simulink model "realtimeE1"  (R2024b)
settings: Solver=FixedStepDiscrete  StartTime=0.0  StopTime=10.0  FixedStep=0.01  RelTol=1e-3  EnableMultiTasking=on
values from neighbouring files (symbols this model uses):
  C = [1,0,0,0]    [S6S10.m]
  CCC = Ts/(Tc+Ts)    [S6S10.m]
undefined symbols (not defined in the file or in its folder): denFd, denH, denHw, DiscIntNeverNeededParam, drv, dspblkCoreblockFVToolHelper, gbox, gcbh, integral, K, numFd, numH, numHw, sens, Ts, wheel
libraries: BalRobTbx_baselib x9
settings Model: ExtModeTrigDuration=2  Creator=lucag  LastModifiedBy=galeazzolu
settings SolverCC: AutoInsertRateTranBlk=on
settings OptimizationCC: EnhancedBackFolding=on  PassReuseOutputArgsAs=Individual arguments  ZeroExternalMemoryAtStartup=off  ZeroInternalMemoryAtStartup=off  MaxStackSize=64  OptimizeBlockOrder=speed  DifferentSizesBufferReuse=on  OptimizationCustomize=off  EfficientTunableParamExpr=on
settings DebuggingCC: ParameterTunabilityLossMsg=error
settings HardwareCC: ProdBitPerInt=16  ProdBitPerPointer=16  ProdBitPerSizeT=16  ProdBitPerPtrDiffT=16  ProdLargestAtomicFloat=None  ProdWordSize=8  ProdHWDeviceType=Atmel->AVR
settings SFSimCC: MATLABDynamicMemAlloc=off
settings RTWCC: Description=Embedded Coder  SystemTargetFile=ert.tlc  HardwareBoard=Arduino Mega 2560  TemplateMakefile=ert_default_tmf  Toolchain=Arduino AVR  BuildConfiguration=Faster Runs
settings CodeAppCC: ForceParamTrailComments=on  IgnoreCustomStorageClasses=off  OperatorAnnotations=on  SimulinkDataObjDesc=on  SFDataObjDesc=on  InsertBlockDesc=on
settings ERTTargetCC: SupportContinuousTime=on  SupportVariableSizeSignals=on  ExtModeTransport=3  ExtModeStaticAlloc=on  ExtModeAutomaticAllocSize=off  ExtModeStaticAllocSize=2048  ExtModeMexFile=ext_xcp  ExtModeIntrfLevel=Level2 - Open  InlinedParameterPlacement=Hierarchical

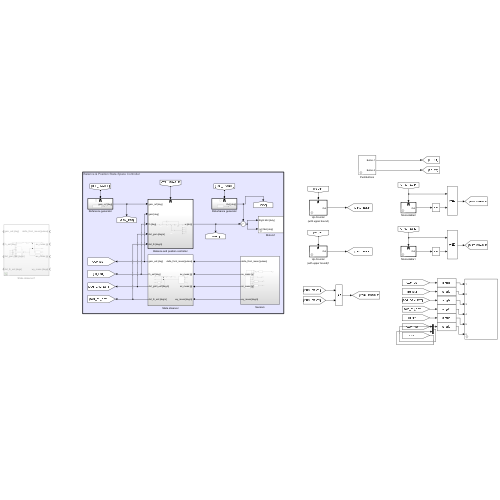
[thumbnail: Simulink's stored preview of the top-level diagram]
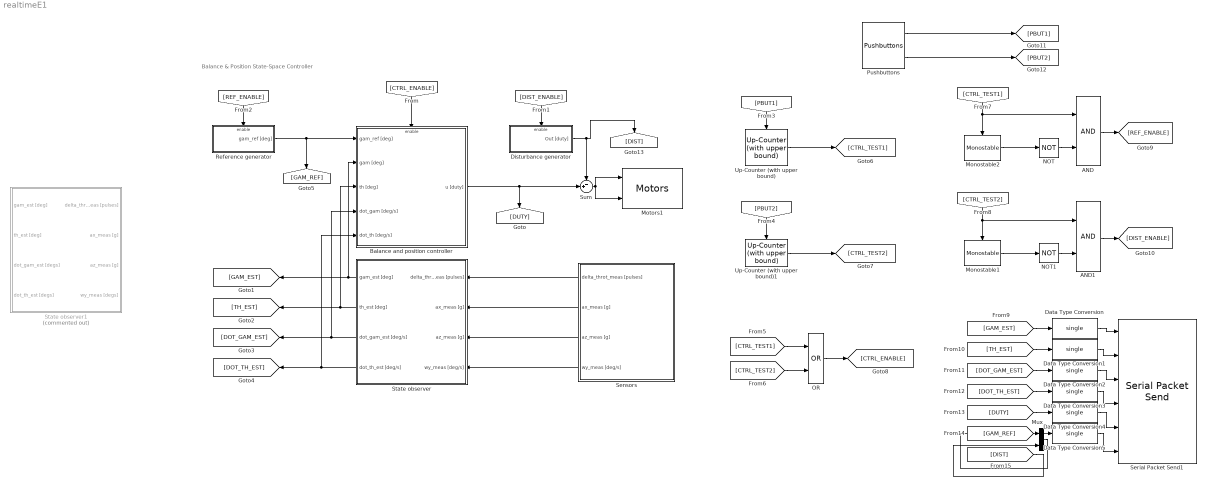
== system realtimeE1 ==
  note: Balance & Position State-Space Controller
  AND : Logic  AllPortsSameDT=off  OutDataTypeStr=boolean
  AND1 : Logic  AllPortsSameDT=off  OutDataTypeStr=boolean
  Balance and position controller : Subsystem  TreatAsAtomicUnit=on
  Data Type Conversion{,1..5} (6 alike) : DataTypeConversion  OutDataTypeStr=single  SaturateOnIntegerOverflow=off  RndMeth=Floor
  Disturbance generator : Subsystem  TreatAsAtomicUnit=on
  Monostable1 : BalRobTbx_baselib/Utilities/Monostable  Tp=13
      settings: SourceProductName=Balancing Robot Toolbox
  Monostable2 : BalRobTbx_baselib/Utilities/Monostable  Tp=10
      settings: SourceProductName=Balancing Robot Toolbox
  Motors1 : BalRobTbx_baselib/Outputs/Motors
      settings: SourceProductName=Balancing Robot Toolbox
  Mux : Mux  Inputs=2
  NOT : Logic  Operator=NOT  AllPortsSameDT=off  OutDataTypeStr=boolean
  NOT1 : Logic  Operator=NOT  AllPortsSameDT=off  OutDataTypeStr=boolean
  OR : Logic  Operator=OR  AllPortsSameDT=off  OutDataTypeStr=boolean
  Pushbuttons : BalRobTbx_baselib/Inputs/Pushbuttons
      settings: SourceProductName=Balancing Robot Toolbox
  Reference generator : Subsystem  TreatAsAtomicUnit=on
  Sensors : Subsystem
  Serial Packet Send1 : BalRobTbx_baselib/Communication/Serial Packet Send  serialLinkOpt=Bluetooth  baudRateOpt=38400  waitHostTxCmd=on  txStartCmd=65  txStopCmd=66  packetSpec={'single', 'single', 'single', 'single', 'single', '2*single'}  cobsEncoded=on  nullTerminated=on  showEnablePort=off
      settings: SourceProductName=Balancing Robot Toolbox
  State observer : Subsystem
  State observer1 : Subsystem  Commented=on
  Sum : Sum  Inputs=-+|
  Up-Counter (with upper bound) : BalRobTbx_baselib/Utilities/Up-Counter (with upper bound)  CMAX=1  C0=0
      settings: SourceProductName=Balancing Robot Toolbox
  Up-Counter (with upper bound)1 : BalRobTbx_baselib/Utilities/Up-Counter (with upper bound)  CMAX=1  C0=0
      settings: SourceProductName=Balancing Robot Toolbox
  wires:
  [CTRL_ENABLE] -> Balance and position controller/Enable
  Balance and position controller/1(u [duty]) -> [DUTY], Sum/2
  Disturbance generator/1(Out [duty]) -> [DIST], Sum/1
  [DIST_ENABLE] -> Disturbance generator/Enable
  Sum/1 -> Motors1/1, Motors1/2
  Sensors/1(delta_throt_meas [pulses]) -> State observer/1(delta_throt_meas [pulses])
  Sensors/2(ax_meas [g]) -> State observer/2(ax_meas [g])
  Sensors/3(az_meas [g]) -> State observer/3(az_meas [g])
  Sensors/4(wy_meas [deg/s]) -> State observer/4(wy_meas [deg/s])
  State observer/1(gam_est [deg]) -> Balance and position controller/2(gam [deg]), [GAM_EST]
  State observer/2(th_est [deg]) -> Balance and position controller/3(th [deg]), [TH_EST]
  State observer/3(dot_gam_est [deg/s]) -> Balance and position controller/4(dot_gam [deg/s]), [DOT_GAM_EST]
  State observer/4(dot_th_est [deg/s]) -> Balance and position controller/5(dot_th [deg/s]), [DOT_TH_EST]
  Reference generator/1(gam_ref [deg]) -> Balance and position controller/1(gam_ref [deg]), [GAM_REF]
  [REF_ENABLE] -> Reference generator/Enable
  [PBUT1] -> Up-Counter (with upper bound)/Trigger
  Up-Counter (with upper bound)/1 -> [CTRL_TEST1]
  Up-Counter (with upper bound)1/1 -> [CTRL_TEST2]
  [PBUT2] -> Up-Counter (with upper bound)1/Trigger
  [CTRL_TEST1] -> OR/1
  [CTRL_TEST2] -> OR/2
  OR/1 -> [CTRL_ENABLE]
  [CTRL_TEST1] -> Monostable2/Enable, AND/1
  Monostable2/1 -> NOT/1
  NOT/1 -> AND/2
  AND/1 -> [REF_ENABLE]
  AND1/1 -> [DIST_ENABLE]
  NOT1/1 -> AND1/2
  Monostable1/1 -> NOT1/1
  Pushbuttons/2 -> [PBUT2]
  Pushbuttons/1 -> [PBUT1]
  [CTRL_TEST2] -> Monostable1/Enable, AND1/1
  [GAM_EST] -> Data Type Conversion/1
  [TH_EST] -> Data Type Conversion1/1
  [DOT_GAM_EST] -> Data Type Conversion2/1
  [DOT_TH_EST] -> Data Type Conversion3/1
  [DUTY] -> Data Type Conversion4/1
  Data Type Conversion5/1 -> Serial Packet Send1/6
  Data Type Conversion4/1 -> Serial Packet Send1/5
  Data Type Conversion3/1 -> Serial Packet Send1/4
  Data Type Conversion2/1 -> Serial Packet Send1/3
  Data Type Conversion1/1 -> Serial Packet Send1/2
  Data Type Conversion/1 -> Serial Packet Send1/1
  [GAM_REF] -> Mux/1
  [DIST] -> Mux/2
  Mux/1 -> Data Type Conversion5/1

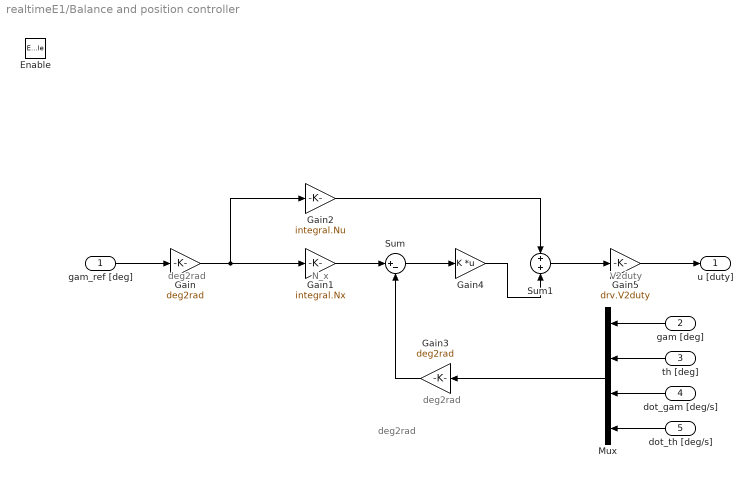
== system realtimeE1/Balance and position controller ==
  note: deg2rad
  note: deg2rad
  note: deg2rad
  note: N_x
  note: V2duty
  gam_ref [deg] : Inport
  gam [deg] : Inport  Port=2
  th [deg] : Inport  Port=3
  dot_gam [deg/s] : Inport  Port=4
  dot_th [deg/s] : Inport  Port=5
  Enable : EnablePort
  Gain : Gain  Gain=deg2rad
  Gain1 : Gain  Gain=integral.Nx
  Gain2 : Gain  Gain=integral.Nu
  Gain3 : Gain  Gain=deg2rad
  Gain4 : Gain  Gain=K  Multiplication=Matrix(K*u)
  Gain5 : Gain  Gain=drv.V2duty
  Mux : Mux
  Sum : Sum  Inputs=|+-
  Sum1 : Sum
  u [duty] : Outport
  wires:
  th [deg]/1 -> Mux/2
  Gain1/1 -> Sum/1
  Gain5/1 -> u [duty]/1
  Gain/1 -> Gain2/1, Gain1/1
  Gain2/1 -> Sum1/1
  Gain3/1 -> Sum/2
  Sum/1 -> Gain4/1
  Mux/1 -> Gain3/1
  Gain4/1 -> Sum1/2
  gam [deg]/1 -> Mux/1
  Sum1/1 -> Gain5/1
  dot_th [deg/s]/1 -> Mux/4
  gam_ref [deg]/1 -> Gain/1
  dot_gam [deg/s]/1 -> Mux/3

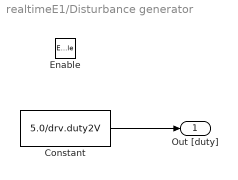
== system realtimeE1/Disturbance generator ==
  Enable : EnablePort
  Constant : Constant  Value=5.0/drv.duty2V
  Out [duty] : Outport  OutputWhenDisabled=reset  InitialOutput=0
  wires:
  Constant/1 -> Out [duty]/1

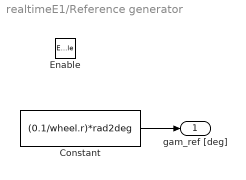
== system realtimeE1/Reference generator ==
  Enable : EnablePort
  Constant : Constant  Value=(0.1/wheel.r)*rad2deg
  gam_ref [deg] : Outport  OutputWhenDisabled=reset  InitialOutput=0
  wires:
  Constant/1 -> gam_ref [deg]/1

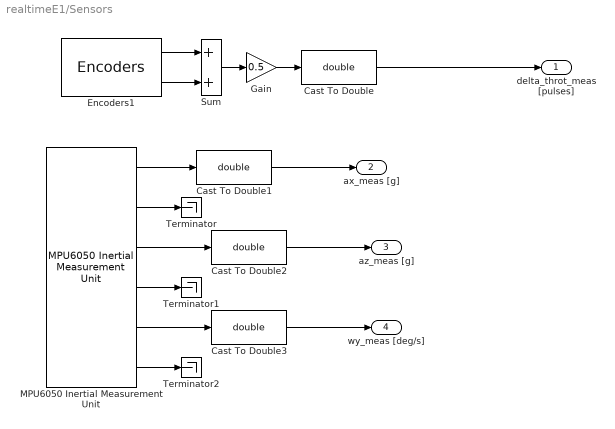
== system realtimeE1/Sensors ==
  Cast To Double{,1..3} (4 alike) : DataTypeConversion  OutDataTypeStr=double  SaturateOnIntegerOverflow=off  RndMeth=Floor
  Encoders1 : BalRobTbx_baselib/Inputs/Encoders
      settings: SourceProductName=Balancing Robot Toolbox
  Gain : Gain  Gain=0.5
  MPU6050 Inertial Measurement Unit : BalRobTbx_baselib/Inputs/MPU6050 Inertial Measurement Unit
      settings: SourceProductName=Balancing Robot Toolbox
  Sum : Sum
  Terminator : Terminator
  Terminator1 : Terminator
  Terminator2 : Terminator
  delta_throt_meas [pulses] : Outport
  ax_meas [g] : Outport  Port=2
  az_meas [g] : Outport  Port=3
  wy_meas [deg/s] : Outport  Port=4
  wires:
  Encoders1/1 -> Sum/1
  Encoders1/2 -> Sum/2
  Sum/1 -> Gain/1
  Gain/1 -> Cast To Double/1
  Cast To Double/1 -> delta_throt_meas [pulses]/1
  MPU6050 Inertial Measurement Unit/1 -> Cast To Double1/1
  MPU6050 Inertial Measurement Unit/3 -> Cast To Double2/1
  MPU6050 Inertial Measurement Unit/5 -> Cast To Double3/1
  MPU6050 Inertial Measurement Unit/2 -> Terminator/1
  MPU6050 Inertial Measurement Unit/4 -> Terminator1/1
  MPU6050 Inertial Measurement Unit/6 -> Terminator2/1
  Cast To Double1/1 -> ax_meas [g]/1
  Cast To Double2/1 -> az_meas [g]/1
  Cast To Double3/1 -> wy_meas [deg/s]/1

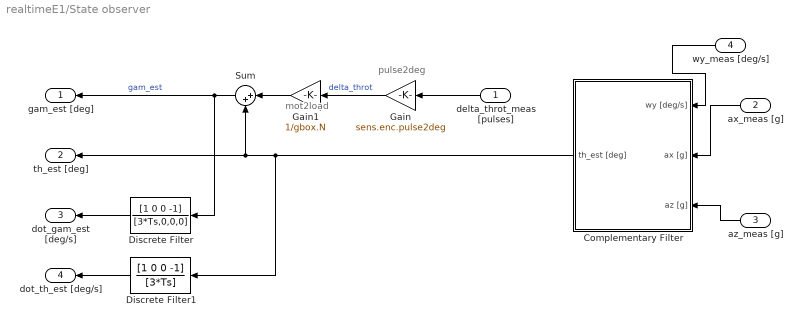
== system realtimeE1/State observer ==
  note: mot2load
  note: pulse2deg
  delta_throt_meas [pulses] : Inport
  ax_meas [g] : Inport  Port=2
  az_meas [g] : Inport  Port=3
  wy_meas [deg/s] : Inport  Port=4
  Complementary Filter : Subsystem
  Discrete Filter : DiscreteFilter  LoadFcn=dspblkCoreblockFVToolHelper(gcbh,'load');  Numerator=[1 0 0 -1]  Denominator=[3*Ts,0,0,0]  SampleTime=Ts
      settings: CopyFcn=dspblkCoreblockFVToolHelper(gcbh,'copy');  DeleteFcn=dspblkCoreblockFVToolHelper(gcbh,'close');  ModelCloseFcn=dspblkCoreblockFVToolHelper(gcbh,'close');  PreSaveFcn=dspblkCoreblockFVToolHelper(gcbh,'presave');  PostSaveFcn=dspblkCoreblockFVToolHelper(gcbh,'postsave');  CloseFcn=dspblkCoreblockFVToolHelper(gcbh,'close');
  Discrete Filter1 : DiscreteFilter  LoadFcn=dspblkCoreblockFVToolHelper(gcbh,'load');  Numerator=[1 0 0 -1]  Denominator=[3*Ts]  SampleTime=Ts
      settings: CopyFcn=dspblkCoreblockFVToolHelper(gcbh,'copy');  DeleteFcn=dspblkCoreblockFVToolHelper(gcbh,'close');  ModelCloseFcn=dspblkCoreblockFVToolHelper(gcbh,'close');  PreSaveFcn=dspblkCoreblockFVToolHelper(gcbh,'presave');  PostSaveFcn=dspblkCoreblockFVToolHelper(gcbh,'postsave');  CloseFcn=dspblkCoreblockFVToolHelper(gcbh,'close');
  Gain : Gain  Gain=sens.enc.pulse2deg
  Gain1 : Gain  Gain=1/gbox.N
  Sum : Sum  Inputs=|++
  gam_est [deg] : Outport
  th_est [deg] : Outport  Port=2
  dot_gam_est [deg/s] : Outport  Port=3
  dot_th_est [deg/s] : Outport  Port=4
  wires:
  Discrete Filter1/1 -> dot_th_est [deg/s]/1
  Sum/1 -> Discrete Filter/1, gam_est [deg]/1  "gam_est"
  Complementary Filter/1(th_est [deg]) -> Discrete Filter1/1, Sum/2, th_est [deg]/1
  Gain1/1 -> Sum/1
  delta_throt_meas [pulses]/1 -> Gain/1
  Discrete Filter/1 -> dot_gam_est [deg/s]/1
  Gain/1 -> Gain1/1  "delta_throt"
  az_meas [g]/1 -> Complementary Filter/3(az [g])
  wy_meas [deg/s]/1 -> Complementary Filter/1(wy [deg/s])
  ax_meas [g]/1 -> Complementary Filter/2(ax [g])

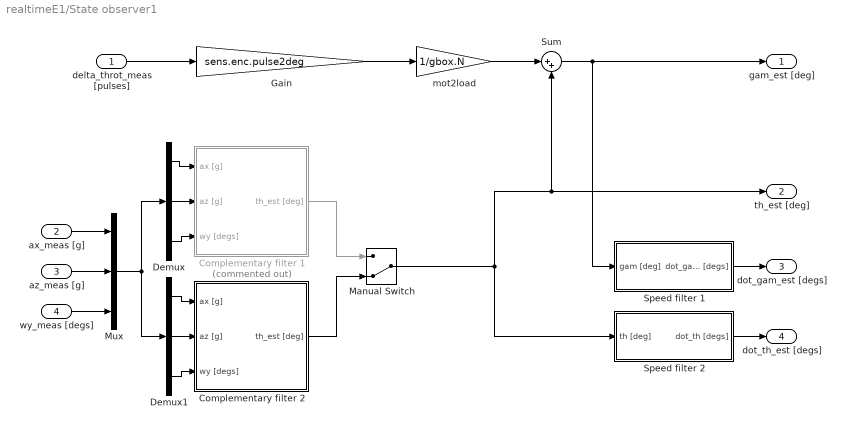
== system realtimeE1/State observer1 ==
  delta_throt_meas [pulses] : Inport
  ax_meas [g] : Inport  Port=2
  az_meas [g] : Inport  Port=3
  wy_meas [degs] : Inport  Port=4
  Complementary filter 1 : Subsystem  Commented=on
  Complementary filter 2 : Subsystem
  Demux : Demux  Outputs=3
  Demux1 : Demux  Outputs=3
  Gain : Gain  Gain=sens.enc.pulse2deg
  Manual Switch : ManualSwitch  CurrentSetting=0
  Mux : Mux  Inputs=3
  Speed filter 1 : Subsystem
  Speed filter 2 : Subsystem
  Sum : Sum  Inputs=|++
  mot2load : Gain  Gain=1/gbox.N
  gam_est [deg] : Outport
  th_est [deg] : Outport  Port=2
  dot_gam_est [degs] : Outport  Port=3
  dot_th_est [degs] : Outport  Port=4
  wires:
  delta_throt_meas [pulses]/1 -> Gain/1
  Gain/1 -> mot2load/1
  mot2load/1 -> Sum/1
  Sum/1 -> Speed filter 1/1(gam [deg]), gam_est [deg]/1
  Speed filter 1/1(dot_gam [degs]) -> dot_gam_est [degs]/1
  Speed filter 2/1(dot_th [degs]) -> dot_th_est [degs]/1
  ax_meas [g]/1 -> Mux/1
  az_meas [g]/1 -> Mux/2
  wy_meas [degs]/1 -> Mux/3
  Demux/1 -> Complementary filter 1/1(ax [g])
  Demux/3 -> Complementary filter 1/3(wy [degs])
  Demux/2 -> Complementary filter 1/2(az [g])
  Demux1/2 -> Complementary filter 2/2(az [g])
  Demux1/1 -> Complementary filter 2/1(ax [g])
  Demux1/3 -> Complementary filter 2/3(wy [degs])
  Mux/1 -> Demux/1, Demux1/1
  Complementary filter 1/1(th_est [deg]) -> Manual Switch/1
  Complementary filter 2/1(th_est [deg]) -> Manual Switch/2
  Manual Switch/1 -> Sum/2, th_est [deg]/1, Speed filter 2/1(th [deg])

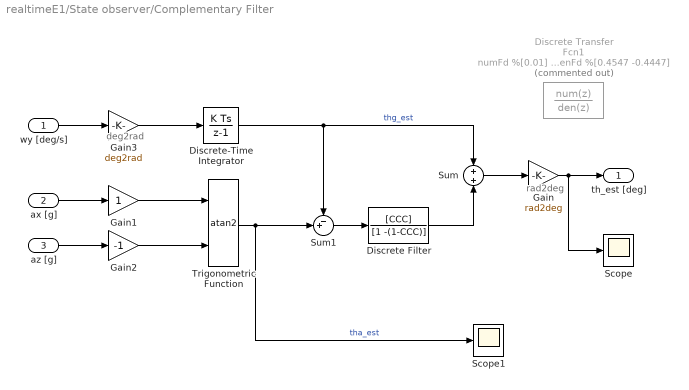
== system realtimeE1/State observer/Complementary Filter ==
  note: rad2deg
  note: deg2rad
  wy [deg/s] : Inport
  ax [g] : Inport  Port=2
  az [g] : Inport  Port=3
  Discrete Transfer Fcn1 : DiscreteTransferFcn  Commented=on  LoadFcn=dspblkCoreblockFVToolHelper(gcbh,'load');  Numerator=numFd %[0.01]  Denominator=denFd %[0.4547 -0.4447]  SampleTime=Ts
      settings: CopyFcn=dspblkCoreblockFVToolHelper(gcbh,'copy');  DeleteFcn=dspblkCoreblockFVToolHelper(gcbh,'close');  ModelCloseFcn=dspblkCoreblockFVToolHelper(gcbh,'close');  PreSaveFcn=dspblkCoreblockFVToolHelper(gcbh,'presave');  PostSaveFcn=dspblkCoreblockFVToolHelper(gcbh,'postsave');  CloseFcn=dspblkCoreblockFVToolHelper(gcbh,'close');
  Discrete Filter : DiscreteFilter  LoadFcn=dspblkCoreblockFVToolHelper(gcbh,'load');  Numerator=[CCC]  Denominator=[1 -(1-CCC)]
      settings: CopyFcn=dspblkCoreblockFVToolHelper(gcbh,'copy');  DeleteFcn=dspblkCoreblockFVToolHelper(gcbh,'close');  ModelCloseFcn=dspblkCoreblockFVToolHelper(gcbh,'close');  PreSaveFcn=dspblkCoreblockFVToolHelper(gcbh,'presave');  PostSaveFcn=dspblkCoreblockFVToolHelper(gcbh,'postsave');  CloseFcn=dspblkCoreblockFVToolHelper(gcbh,'close');
  Discrete-Time Integrator : DiscreteIntegrator  SampleTime=Ts  ICPrevOutput=DiscIntNeverNeededParam  ICPrevScaledInput=DiscIntNeverNeededParam
  Gain : Gain  Gain=rad2deg
  Gain1 : Gain
  Gain2 : Gain  Gain=-1
  Gain3 : Gain  Gain=deg2rad
  Scope : Scope
  Scope1 : Scope
  Sum : Sum  Inputs=+|+
  Sum1 : Sum  Inputs=-+|
  Trigonometric Function : Trigonometry  Operator=atan2
  th_est [deg] : Outport
  wires:
  Sum/1 -> Gain/1
  ax [g]/1 -> Gain1/1
  Gain1/1 -> Trigonometric Function/1
  az [g]/1 -> Gain2/1
  Gain2/1 -> Trigonometric Function/2
  wy [deg/s]/1 -> Gain3/1
  Gain3/1 -> Discrete-Time Integrator/1
  Trigonometric Function/1 -> Scope1/1, Sum1/2  "tha_est"
  Discrete-Time Integrator/1 -> Sum/1, Sum1/1  "thg_est"
  Sum1/1 -> Discrete Filter/1
  Discrete Filter/1 -> Sum/2
  Gain/1 -> Scope/1, th_est [deg]/1

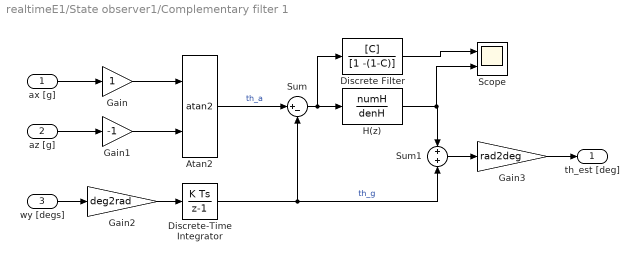
== system realtimeE1/State observer1/Complementary filter 1 ==
  ax [g] : Inport
  az [g] : Inport  Port=2
  wy [degs] : Inport  Port=3
  Atan2 : Trigonometry  Operator=atan2
  Discrete Filter : DiscreteFilter  LoadFcn=dspblkCoreblockFVToolHelper(gcbh,'load');  Numerator=[C]  Denominator=[1 -(1-C)]
      settings: CopyFcn=dspblkCoreblockFVToolHelper(gcbh,'copy');  DeleteFcn=dspblkCoreblockFVToolHelper(gcbh,'close');  ModelCloseFcn=dspblkCoreblockFVToolHelper(gcbh,'close');  PreSaveFcn=dspblkCoreblockFVToolHelper(gcbh,'presave');  PostSaveFcn=dspblkCoreblockFVToolHelper(gcbh,'postsave');  CloseFcn=dspblkCoreblockFVToolHelper(gcbh,'close');
  Discrete-Time Integrator : DiscreteIntegrator  SampleTime=Ts  ICPrevOutput=DiscIntNeverNeededParam  ICPrevScaledInput=DiscIntNeverNeededParam
  Gain : Gain
  Gain1 : Gain  Gain=-1
  Gain2 : Gain  Gain=deg2rad
  Gain3 : Gain  Gain=rad2deg
  H(z) : DiscreteTransferFcn  Numerator=numH  Denominator=denH
  Scope : Scope  NumInputPorts=2
  Sum : Sum  Inputs=|+-
  Sum1 : Sum  Inputs=+|+
  th_est [deg] : Outport
  wires:
  ax [g]/1 -> Gain/1
  az [g]/1 -> Gain1/1
  Gain/1 -> Atan2/1
  Gain1/1 -> Atan2/2
  Atan2/1 -> Sum/1  "th_a"
  wy [degs]/1 -> Gain2/1
  Gain2/1 -> Discrete-Time Integrator/1
  Discrete-Time Integrator/1 -> Sum1/2, Sum/2  "th_g"
  Sum/1 -> Discrete Filter/1, H(z)/1
  H(z)/1 -> Scope/2, Sum1/1
  Sum1/1 -> Gain3/1
  Gain3/1 -> th_est [deg]/1
  Discrete Filter/1 -> Scope/1

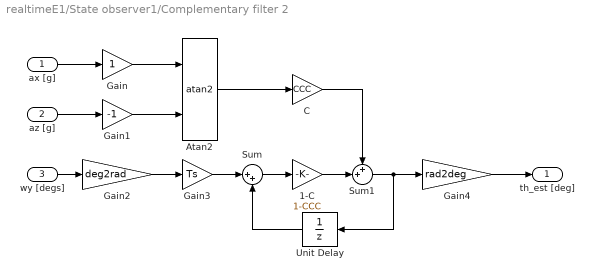
== system realtimeE1/State observer1/Complementary filter 2 ==
  ax [g] : Inport
  az [g] : Inport  Port=2
  wy [degs] : Inport  Port=3
  1-C : Gain  Gain=1-CCC
  Atan2 : Trigonometry  Operator=atan2
  C : Gain  Gain=CCC
  Gain : Gain
  Gain1 : Gain  Gain=-1
  Gain2 : Gain  Gain=deg2rad
  Gain3 : Gain  Gain=Ts
  Gain4 : Gain  Gain=rad2deg
  Sum : Sum  Inputs=|++
  Sum1 : Sum  Inputs=++|
  Unit Delay : UnitDelay  SampleTime=-1  HasFrameUpgradeWarning=on
  th_est [deg] : Outport
  wires:
  Gain/1 -> Atan2/1
  az [g]/1 -> Gain1/1
  Gain1/1 -> Atan2/2
  ax [g]/1 -> Gain/1
  Atan2/1 -> C/1
  wy [degs]/1 -> Gain2/1
  Gain2/1 -> Gain3/1
  Gain3/1 -> Sum/1
  Sum/1 -> 1-C/1
  C/1 -> Sum1/1
  1-C/1 -> Sum1/2
  Sum1/1 -> Unit Delay/1, Gain4/1
  Unit Delay/1 -> Sum/2
  Gain4/1 -> th_est [deg]/1

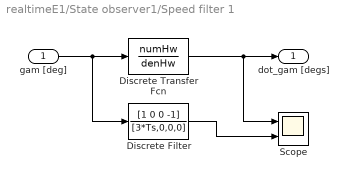
== system realtimeE1/State observer1/Speed filter 1 ==
  gam [deg] : Inport
  Discrete Transfer Fcn : DiscreteTransferFcn  LoadFcn=dspblkCoreblockFVToolHelper(gcbh,'load');  Numerator=numHw  Denominator=denHw
      settings: CopyFcn=dspblkCoreblockFVToolHelper(gcbh,'copy');  DeleteFcn=dspblkCoreblockFVToolHelper(gcbh,'close');  ModelCloseFcn=dspblkCoreblockFVToolHelper(gcbh,'close');  PreSaveFcn=dspblkCoreblockFVToolHelper(gcbh,'presave');  PostSaveFcn=dspblkCoreblockFVToolHelper(gcbh,'postsave');  CloseFcn=dspblkCoreblockFVToolHelper(gcbh,'close');
  Discrete Filter : DiscreteFilter  LoadFcn=dspblkCoreblockFVToolHelper(gcbh,'load');  Numerator=[1 0 0 -1]  Denominator=[3*Ts,0,0,0]  SampleTime=Ts
      settings: CopyFcn=dspblkCoreblockFVToolHelper(gcbh,'copy');  DeleteFcn=dspblkCoreblockFVToolHelper(gcbh,'close');  ModelCloseFcn=dspblkCoreblockFVToolHelper(gcbh,'close');  PreSaveFcn=dspblkCoreblockFVToolHelper(gcbh,'presave');  PostSaveFcn=dspblkCoreblockFVToolHelper(gcbh,'postsave');  CloseFcn=dspblkCoreblockFVToolHelper(gcbh,'close');
  Scope : Scope  NumInputPorts=2
  dot_gam [degs] : Outport
  wires:
  gam [deg]/1 -> Discrete Filter/1, Discrete Transfer Fcn/1
  Discrete Transfer Fcn/1 -> Scope/1, dot_gam [degs]/1
  Discrete Filter/1 -> Scope/2

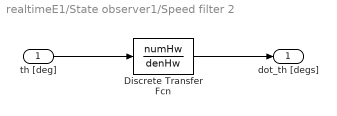
== system realtimeE1/State observer1/Speed filter 2 ==
  th [deg] : Inport
  Discrete Transfer Fcn : DiscreteTransferFcn  LoadFcn=dspblkCoreblockFVToolHelper(gcbh,'load');  Numerator=numHw  Denominator=denHw
      settings: CopyFcn=dspblkCoreblockFVToolHelper(gcbh,'copy');  DeleteFcn=dspblkCoreblockFVToolHelper(gcbh,'close');  ModelCloseFcn=dspblkCoreblockFVToolHelper(gcbh,'close');  PreSaveFcn=dspblkCoreblockFVToolHelper(gcbh,'presave');  PostSaveFcn=dspblkCoreblockFVToolHelper(gcbh,'postsave');  CloseFcn=dspblkCoreblockFVToolHelper(gcbh,'close');
  dot_th [degs] : Outport
  wires:
  th [deg]/1 -> Discrete Transfer Fcn/1
  Discrete Transfer Fcn/1 -> dot_th [degs]/1
